simulink model "logo_integration_task"  (Simulink 3.00)
libraries: lib x12, mathlib x7, logiclib x3, genlib x1

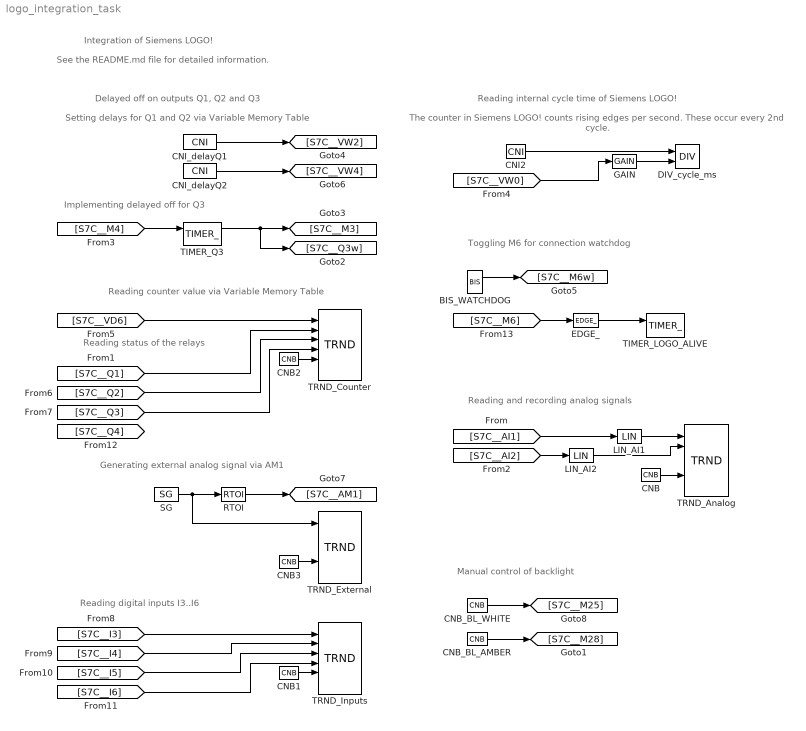
== system logo_integration_task ==
  note: Delayed off on outputs Q1, Q2 and Q3
  note: Setting delays for Q1 and Q2 via Variable Memory Table
  note: Implementing delayed off for Q3
  note: Toggling M6 for connection watchdog
  note: Generating external analog signal via AM1
  note: Reading internal cycle time of Siemens LOGO!
  note: Reading counter value via Variable Memory Table
  note: Reading status of the relays
  note: The counter in Siemens LOGO! counts rising edges per second. These
      | occur every 2nd cycle.
  note: Reading and recording analog signals
  note: Reading digital inputs I3..I6
  note: Manual control of backlight
  note: Integration of Siemens LOGO!
  note: See the README.md file for detailed information.
  BIS_WATCHDOG : genlib/BIS  Y0=off  t1=0.1  t2=0.2  t3=0  t4=4  t5=5  t6=6  t7=7  t8=8  RPT=on  bEdit=off
  CNB{,1..3} (4 alike) : lib/CNB  YCN=on
  CNB_BL_AMBER : lib/CNB  YCN=off
  CNB_BL_WHITE : lib/CNB  YCN=off
  CNI2 : mathlib/CNI  icn=1
  CNI_delayQ1 : mathlib/CNI  icn=100
  CNI_delayQ2 : mathlib/CNI  icn=200
  DIV_cycle_ms : mathlib/DIV  yerr=0
  EDGE_ : logiclib/EDGE_  iedge=3: Both edges
  GAIN : mathlib/GAIN  k=0.002
  LIN_AI1 : mathlib/LIN  u1=0  y1=0  u2=1000  y2=10
  LIN_AI2 : mathlib/LIN  u1=0  y1=0  u2=1000  y2=10
  RTOI : lib/RTOI
  SG : lib/SG  isig=1: SINE  amp=500  freq=0.1  phase=0.0000000E+000  offset=0  ifrunit=1: Hz  iphunit=1: degrees
  TIMER_LOGO_ALIVE : logiclib/TIMER_  mode=3: Delayed OFF  pt=0.5
  TIMER_Q3 : logiclib/TIMER_  mode=1: Pulse generator  pt=3
  TRND_Analog : lib/TRND  n=2  l=9000  btype=8: Double  ptype1=1: Store  ptype2=1: Store  ptype3=1: Store  ptype4=1: Store  pfac=1  afac=0  arc=0  id=2  Title=Analog signals  timesrc=1
  TRND_Counter : lib/TRND  n=4  l=9000  btype=8: Double  ptype1=1: Store  ptype2=1: Store  ptype3=1: Store  ptype4=1: Store  pfac=1  afac=0  arc=0  id=1  Title=Counter  timesrc=1
  TRND_External : lib/TRND  n=1  l=9000  btype=8: Double  ptype1=1: Store  ptype2=1: Store  ptype3=1: Store  ptype4=1: Store  pfac=1  afac=0  arc=0  id=1  Title=External analog signal  timesrc=1: CORETIMER
  TRND_Inputs : lib/TRND  n=4  l=9000  btype=8: Double  ptype1=1: Store  ptype2=1: Store  ptype3=1: Store  ptype4=1: Store  pfac=1  afac=0  arc=0  id=3  Title=Digital inputs I3, I4, I5, I6  timesrc=1
  wires:
  BIS_WATCHDOG/1 -> [S7C__M6w]
  CNB/1 -> TRND_Analog/5
  CNB1/1 -> TRND_Inputs/5
  CNB2/1 -> TRND_Counter/5
  CNB3/1 -> TRND_External/5
  CNB_BL_AMBER/1 -> [S7C__M28]
  CNB_BL_WHITE/1 -> [S7C__M25]
  CNI2/1 -> DIV_cycle_ms/1
  CNI_delayQ1/1 -> [S7C__VW2]
  CNI_delayQ2/1 -> [S7C__VW4]
  EDGE_/1 -> TIMER_LOGO_ALIVE/1
  [S7C__AI1] -> LIN_AI1/1
  [S7C__Q1] -> TRND_Counter/2
  [S7C__I5] -> TRND_Inputs/3
  [S7C__I6] -> TRND_Inputs/4
  [S7C__M6] -> EDGE_/1
  [S7C__AI2] -> LIN_AI2/1
  [S7C__M4] -> TIMER_Q3/1
  [S7C__VW0] -> GAIN/1
  [S7C__VD6] -> TRND_Counter/1
  [S7C__Q2] -> TRND_Counter/3
  [S7C__Q3] -> TRND_Counter/4
  [S7C__I3] -> TRND_Inputs/1
  [S7C__I4] -> TRND_Inputs/2
  GAIN/1 -> DIV_cycle_ms/2
  LIN_AI1/1 -> TRND_Analog/1
  LIN_AI2/1 -> TRND_Analog/2
  RTOI/1 -> [S7C__AM1]
  SG/1 -> RTOI/1, TRND_External/1
  TIMER_Q3/1 -> [S7C__Q3w], [S7C__M3]
